simulink model "Ctrl_For_HRV_20260625"  (R2024b)
settings: Solver=ode4  StartTime=0.0  StopTime=22  FixedStep=0.02  RelTol=1e-3
InitFcn:
  | Parameter;
undefined symbols (not defined in the file or in its folder): CCI_DUI_AngleRate_Controller, CCI_DUI_FlowAngle_Controller, fhan, h_alpha, h_beta, h_miu, h_p, h_q, h_r, PNG_2026_6_23, r_alpha, r_beta, r_miu, r_p, r_q, r_r, xishu, xishu_D_0, xishu_L_0, xishu_l_0, xishu_m_0, xishu_n_0, xishu_Y_0
libraries: simulink x60
(part 2 of 8)

== system Ctrl_For_HRV_20260625/Vehicle_1/FlowAngle_Controller_v1 ==
  alpha_d : Inport
  beta_d : Inport  Port=2
  miu_d : Inport  Port=3
  Demux : Demux  Outputs=9
  From12 : From  Commented=on  GotoTag=dot_alpha_c  TagVisibility=global
  From13 : From  Commented=on  GotoTag=dot_beta_c  TagVisibility=global
  From14 : From  Commented=on  GotoTag=dot_miu_c  TagVisibility=global
  Goto6 : Goto  Commented=on  GotoTag=ddot_alpha_c  TagVisibility=global
  Goto7 : Goto  Commented=on  GotoTag=ddot_beta_c  TagVisibility=global
  Goto8 : Goto  Commented=on  GotoTag=ddot_miu_c  TagVisibility=global
  Interpreted MATLAB Function : MATLABFcn  MATLABFcn=CCI_DUI_FlowAngle_Controller(u(1),u(2),u(3),u(4),u(5),u(6),u(7),u(8),u(9),u(10),u(11),u(12),u(13),u(14),u(15),u(16),u(17),u(18))  OutputDimensions=9
  Mux : Mux  Inputs=18
  Mux1 : Mux  Inputs=3
  Mux2 : Mux  Inputs=3
  Scope_CCI_FlowAngle : Scope
  Scope_DUI_FlowAngle : Scope
  Scope_alpha_d : Scope
  Scope_beta_d : Scope
  Scope_miu_d : Scope
  TD_alpha : Subsystem
  TD_alpha2 : Subsystem
  TD_alpha3 : Subsystem  Commented=on
  TD_alpha4 : Subsystem  Commented=on
  TD_beta : Subsystem
  TD_beta1 : Subsystem
  TD_beta2 : Subsystem
  TD_dotalpha1 : Subsystem  Commented=on
  TD_miu : Subsystem
  p_d : Outport
  q_d : Outport  Port=2
  r_d : Outport  Port=3
  tag scope: alpha_c_v1=global, beta_c_v1=global, dot_alpha_c_v1=global, dot_beta_c_v1=global, dot_miu_c_v1=global, miu_c_v1=global
  wires:
  Demux/7 -> Mux2/1
  Demux/9 -> Mux2/3
  Demux/8 -> Mux2/2
  Mux2/1 -> Scope_DUI_FlowAngle/1
  Mux1/1 -> Scope_CCI_FlowAngle/1
  Demux/6 -> Mux1/3
  Demux/5 -> Mux1/2
  Demux/4 -> Mux1/1
  TD_alpha/1(alpha_c) -> Mux/13, [alpha_c_v1]
  TD_alpha4/1(ddot_miu_c) -> Goto8/1
  From14/1 -> TD_alpha4/1(dot_miu_c)
  TD_alpha3/1(ddot_beta_c) -> Goto7/1
  From13/1 -> TD_alpha3/1(dot_beta_c)
  TD_dotalpha1/1(ddot_alpha_c) -> Goto6/1
  From12/1 -> TD_dotalpha1/1(dot_alpha_c)
  [phi_miu_hat_v1] -> Mux/12
  [phi_beta_hat_v1] -> Mux/11
  [phi_alpha_hat_v1] -> Mux/10
  TD_miu/2(miu_c_dot) -> Mux/18, [dot_miu_c_v1]
  TD_miu/1(miu_c) -> Mux/17, [miu_c_v1]
  miu_d/1 -> TD_miu/1(miu_d), Scope_miu_d/1
  TD_beta/2(beta_c_dot) -> Mux/16, [dot_beta_c_v1]
  TD_beta/1(beta_c) -> Mux/15, [beta_c_v1]
  beta_d/1 -> TD_beta/1(beta_d), Scope_beta_d/1
  TD_alpha/2(alpha_c_dot) -> [dot_alpha_c_v1], Mux/14
  alpha_d/1 -> TD_alpha/1(alpha_d), Scope_alpha_d/1
  Demux/3 -> r_d/1
  Demux/2 -> q_d/1
  Demux/1 -> p_d/1
  Interpreted MATLAB Function/1 -> Demux/1
  Mux/1 -> Interpreted MATLAB Function/1
  [theta_v1] -> Mux/9
  [delta_a_v1] -> Mux/6
  [delta_e_v1] -> Mux/7
  [delta_r_v1] -> Mux/8
  [miu_noise_v1] -> Mux/5
  [beta_noise_v1] -> Mux/4
  [alpha_noise_v1] -> Mux/3
  [V_v1] -> Mux/2
  [H_v1] -> Mux/1

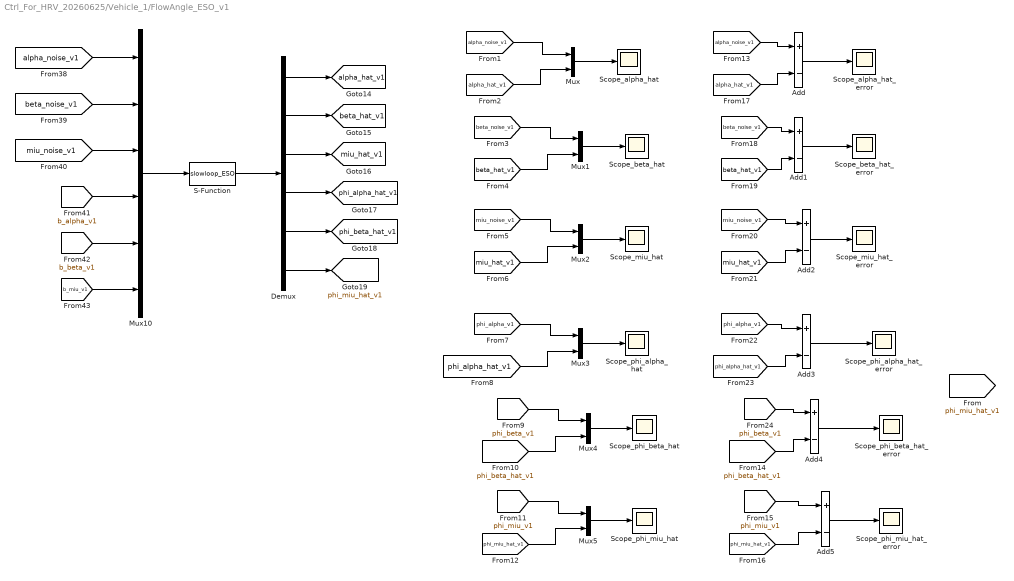
== system Ctrl_For_HRV_20260625/Vehicle_1/FlowAngle_ESO_v1 ==
  Add{,1..5} (6 alike) : Sum  Inputs=+-
  Demux : Demux  Outputs=6
  Mux{,1..5} (6 alike) : Mux  Inputs=2
  Mux10 : Mux  Inputs=6
  S-Function : S-Function  FunctionName=slowloop_ESO  SFunctionDeploymentMode=off  EnableBusSupport=off
  Scope_alpha_hat : Scope
  Scope_alpha_hat_error : Scope
  Scope_beta_hat : Scope
  Scope_beta_hat_error : Scope
  Scope_miu_hat : Scope
  Scope_miu_hat_error : Scope
  Scope_phi_alpha_hat : Scope
  Scope_phi_alpha_hat_error : Scope
  Scope_phi_beta_hat : Scope
  Scope_phi_beta_hat_error : Scope
  Scope_phi_miu_hat : Scope
  Scope_phi_miu_hat_error : Scope
  tag scope: alpha_hat_v1=global, beta_hat_v1=global, miu_hat_v1=global, phi_alpha_hat_v1=global, phi_beta_hat_v1=global, phi_miu_hat_v1=global
  wires:
  [phi_miu_hat_v1] -> Add5/2
  [phi_miu_v1] -> Add5/1
  Add5/1 -> Scope_phi_miu_hat_error/1
  Add4/1 -> Scope_phi_beta_hat_error/1
  [phi_beta_hat_v1] -> Add4/2
  [phi_beta_v1] -> Add4/1
  Add3/1 -> Scope_phi_alpha_hat_error/1
  [phi_alpha_hat_v1] -> Add3/2
  [phi_alpha_v1] -> Add3/1
  Add2/1 -> Scope_miu_hat_error/1
  [miu_hat_v1] -> Add2/2
  [miu_noise_v1] -> Add2/1
  Add1/1 -> Scope_beta_hat_error/1
  [beta_hat_v1] -> Add1/2
  [beta_noise_v1] -> Add1/1
  Add/1 -> Scope_alpha_hat_error/1
  [alpha_hat_v1] -> Add/2
  [alpha_noise_v1] -> Add/1
  Mux3/1 -> Scope_phi_alpha_hat/1
  [phi_alpha_v1] -> Mux3/1
  [phi_alpha_hat_v1] -> Mux3/2
  [phi_beta_v1] -> Mux4/1
  [phi_beta_hat_v1] -> Mux4/2
  Mux4/1 -> Scope_phi_beta_hat/1
  [phi_miu_v1] -> Mux5/1
  [phi_miu_hat_v1] -> Mux5/2
  Mux5/1 -> Scope_phi_miu_hat/1
  Mux2/1 -> Scope_miu_hat/1
  [miu_hat_v1] -> Mux2/2
  [miu_noise_v1] -> Mux2/1
  Mux1/1 -> Scope_beta_hat/1
  [beta_hat_v1] -> Mux1/2
  [beta_noise_v1] -> Mux1/1
  [alpha_hat_v1] -> Mux/2
  [alpha_noise_v1] -> Mux/1
  Mux/1 -> Scope_alpha_hat/1
  [b_miu_v1] -> Mux10/6
  [alpha_noise_v1] -> Mux10/1
  Demux/6 -> [phi_miu_hat_v1]
  Mux10/1 -> S-Function/1
  Demux/4 -> [phi_alpha_hat_v1]
  Demux/3 -> [miu_hat_v1]
  Demux/1 -> [alpha_hat_v1]
  Demux/5 -> [phi_beta_hat_v1]
  S-Function/1 -> Demux/1
  [b_alpha_v1] -> Mux10/4
  Demux/2 -> [beta_hat_v1]
  [beta_noise_v1] -> Mux10/2
  [miu_noise_v1] -> Mux10/3
  [b_beta_v1] -> Mux10/5

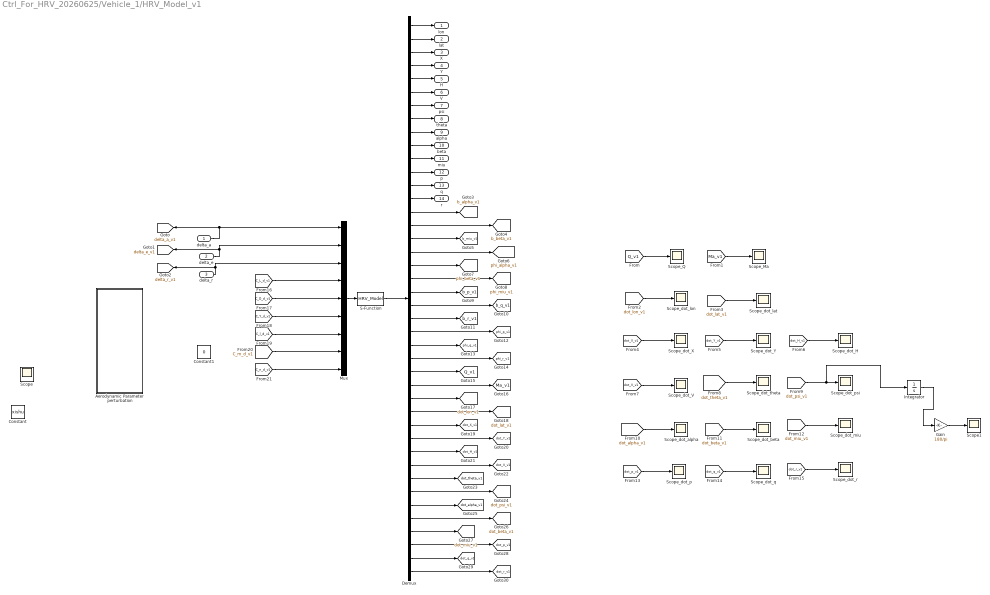
== system Ctrl_For_HRV_20260625/Vehicle_1/HRV_Model_v1 ==
  delta_a : Inport
  delta_e : Inport  Port=2
  delta_r : Inport  Port=3
  Aerodynamic Parameter perturbation : Subsystem
  Constant : Constant  Value=xishu  SampleTime=-1
  Constant1 : Constant  Value=0
  Demux : Demux  Outputs=14 + 12 + 2 + 14
  Gain : Gain  Gain=180/pi
  Integrator : Integrator  InitialCondition=[0 0 -900 -700 0 0 -0.0698131700797732 0 0 0 0 0 0 0 0 0 0 0 0 0 0 0 0 0 0 0 0 0 0 0 0 0 0 0 0 0 0 0 0 0 0 0]
  Mux : Mux  Inputs=9
  S-Function : S-Function  FunctionName=HRV_Model  SFunctionDeploymentMode=off  EnableBusSupport=off
  Scope : Scope
  Scope1 : Scope
  Scope_Ma : Scope
  Scope_Q : Scope
  Scope_dot_H : Scope
  Scope_dot_V : Scope
  Scope_dot_X : Scope
  Scope_dot_Y : Scope
  Scope_dot_alpha : Scope
  Scope_dot_beta : Scope
  Scope_dot_lat : Scope
  Scope_dot_lon : Scope
  Scope_dot_miu : Scope
  Scope_dot_p : Scope
  Scope_dot_psi : Scope
  Scope_dot_q : Scope
  Scope_dot_r : Scope
  Scope_dot_theta : Scope
  lon : Outport
  lat : Outport  Port=2
  X : Outport  Port=3
  Y : Outport  Port=4
  H : Outport  Port=5
  V : Outport  Port=6
  psi : Outport  Port=7
  theta : Outport  Port=8
  alpha : Outport  Port=9
  beta : Outport  Port=10
  miu : Outport  Port=11
  p : Outport  Port=12
  q : Outport  Port=13
  r : Outport  Port=14
  tag scope: Ma_v1=global, Q_v1=global, b_alpha_v1=global, b_beta_v1=global, b_miu_v1=global, b_p_v1=global, b_q_v1=global, b_r_v1=global, delta_a_v1=global, delta_e_v1=global, delta_r_v1=global, dot_H_v1=global, dot_V_v1=global, dot_X_v1=global, dot_Y_v1=global, dot_alpha_v1=global, dot_beta_v1=global, dot_lat_v1=global, dot_lon_v1=global, dot_miu_v1=global, dot_p_v1=global, dot_psi_v1=global, dot_q_v1=global, dot_r_v1=global, dot_theta_v1=global, phi_alpha_v1=global, phi_beta_v1=global, phi_miu_v1=global, phi_p_v1=global, phi_q_v1=global, phi_r_v1=global
  wires:
  Gain/1 -> Scope1/1
  Integrator/1 -> Gain/1
  [C_n_d_v1] -> Mux/9
  [C_m_d_v1] -> Mux/8
  [C_l_d_v1] -> Mux/7
  [C_Y_d_v1] -> Mux/6
  [C_D_d_v1] -> Mux/5
  [C_L_d_v1] -> Mux/4
  [dot_p_v1] -> Scope_dot_p/1
  [dot_q_v1] -> Scope_dot_q/1
  [dot_r_v1] -> Scope_dot_r/1
  [dot_miu_v1] -> Scope_dot_miu/1
  [dot_beta_v1] -> Scope_dot_beta/1
  [dot_alpha_v1] -> Scope_dot_alpha/1
  [dot_psi_v1] -> Scope_dot_psi/1, Integrator/1
  [dot_theta_v1] -> Scope_dot_theta/1
  [dot_V_v1] -> Scope_dot_V/1
  [dot_H_v1] -> Scope_dot_H/1
  [dot_Y_v1] -> Scope_dot_Y/1
  [dot_X_v1] -> Scope_dot_X/1
  [dot_lat_v1] -> Scope_dot_lat/1
  [dot_lon_v1] -> Scope_dot_lon/1
  [Ma_v1] -> Scope_Ma/1
  [Q_v1] -> Scope_Q/1
  Demux/42 -> [dot_r_v1]
  Demux/41 -> [dot_q_v1]
  Demux/40 -> [dot_p_v1]
  Demux/38 -> [dot_beta_v1]
  Demux/39 -> [dot_miu_v1]
  Demux/33 -> [dot_H_v1]
  Demux/35 -> [dot_theta_v1]
  Demux/34 -> [dot_V_v1]
  Demux/36 -> [dot_psi_v1]
  Demux/37 -> [dot_alpha_v1]
  Demux/32 -> [dot_Y_v1]
  Demux/31 -> [dot_X_v1]
  Demux/29 -> [dot_lon_v1]
  Demux/30 -> [dot_lat_v1]
  Demux/28 -> [Ma_v1]
  Demux/27 -> [Q_v1]
  Demux/26 -> [phi_r_v1]
  Demux/25 -> [phi_q_v1]
  Demux/24 -> [phi_p_v1]
  Demux/23 -> [b_r_v1]
  Demux/19 -> [phi_beta_v1]
  Demux/20 -> [phi_miu_v1]
  Demux/22 -> [b_q_v1]
  Demux/21 -> [b_p_v1]
  Demux/17 -> [b_miu_v1]
  Demux/18 -> [phi_alpha_v1]
  Demux/16 -> [b_beta_v1]
  Demux/15 -> [b_alpha_v1]
  Demux/4 -> Y/1
  delta_a/1 -> Mux/1, [delta_a_v1]
  Demux/13 -> q/1
  delta_r/1 -> Mux/3, [delta_r_v1]
  Demux/14 -> r/1
  Demux/6 -> V/1
  delta_e/1 -> Mux/2, [delta_e_v1]
  Demux/5 -> H/1
  Demux/12 -> p/1
  Demux/9 -> alpha/1
  Demux/10 -> beta/1
  Demux/11 -> miu/1
  Demux/7 -> psi/1
  Demux/3 -> X/1
  Demux/2 -> lat/1
  Demux/1 -> lon/1
  S-Function/1 -> Demux/1
  Mux/1 -> S-Function/1
  Demux/8 -> theta/1

== system Ctrl_For_HRV_20260625/Vehicle_1/PNG ==
  Delay : Delay  DelayLength=1
  Demux : Demux  Outputs=3
  MATLAB Function : MATLAB Function  TreatAsAtomicUnit=on
  MATLAB Function1 : MATLAB Function  TreatAsAtomicUnit=on  SystemSampleTime=0.02
  MATLAB Function2 : MATLAB Function  TreatAsAtomicUnit=on
  Mux : Mux  Inputs=7+2
  PNG : MATLABFcn  MATLABFcn=PNG_2026_6_23(u)  OutputDimensions=3
  Scope{,1..4} (5 alike) : Scope
  Scope5 : Scope  NumInputPorts=2
  tag scope: alpha_cmd=global, f_psi=global, miu_cmd=global
  wires:
  Delay/1 -> MATLAB Function1/6(miu_last)
  [theta] -> Mux/9
  [f_psi] -> Mux/8
  MATLAB Function2/1(f_psi) -> [f_psi]
  [H] -> MATLAB Function2/5(H)
  [lat] -> MATLAB Function2/4(lat)
  [psi] -> MATLAB Function2/3(psi)
  [theta] -> MATLAB Function2/2(theta)
  [V] -> MATLAB Function2/1(V)
  Demux/3 -> Scope5/1
  [Q] -> Mux/7
  MATLAB Function1/2(miu_cmd) -> [miu_cmd], Scope3/1, Delay/1
  MATLAB Function1/1(alpha_cmd) -> [alpha_cmd], Scope2/1
  [Ma] -> MATLAB Function1/5(Ma)
  [H] -> MATLAB Function1/4(H)
  [Q] -> MATLAB Function1/3(Q)
  [nz_cmd] -> MATLAB Function1/2(nz_cmd)
  [ny_cmd] -> MATLAB Function1/1(ny_cmd)
  [nz_cmd] -> Scope1/1
  [ny_cmd] -> Scope/1
  Demux/2 -> [nz_cmd], Scope5/2
  Demux/1 -> [ny_cmd]
  PNG/1 -> Demux/1
  [V_target] -> Mux/6
  [Position_target] -> Mux/5
  MATLAB Function/1(v) -> Mux/4, Scope4/1
  [psi] -> MATLAB Function/3(psi)
  [theta] -> MATLAB Function/2(theta)
  [V] -> MATLAB Function/1(V)
  [H] -> Mux/3
  [Y] -> Mux/2
  [X] -> Mux/1
  Mux/1 -> PNG/1

== system Ctrl_For_HRV_20260625/Vehicle_1/actuator1_v1 ==
  delta_e_d : Inport
  Gain : Gain  Gain=50
  Integrator : Integrator
  Saturation : Saturate  UpperLimit=90  LowerLimit=-90
  Saturation1 : Saturate  UpperLimit=30  LowerLimit=-30
  Sum : Sum  Inputs=|+-
  delta_e : Outport
  wires:
  Saturation/1 -> Integrator/1
  Sum/1 -> Gain/1
  Integrator/1 -> Saturation1/1, Sum/2
  delta_e_d/1 -> Sum/1
  Gain/1 -> Saturation/1
  Saturation1/1 -> delta_e/1

== system Ctrl_For_HRV_20260625/Vehicle_1/actuator2_v1 ==
  delta_r_d : Inport
  Gain : Gain  Gain=50
  Integrator : Integrator
  Saturation : Saturate  UpperLimit=90  LowerLimit=-90
  Saturation1 : Saturate  UpperLimit=30  LowerLimit=-30
  Sum : Sum  Inputs=|+-
  delta_r : Outport
  wires:
  Saturation1/1 -> delta_r/1
  Gain/1 -> Saturation/1
  delta_r_d/1 -> Sum/1
  Integrator/1 -> Sum/2, Saturation1/1
  Sum/1 -> Gain/1
  Saturation/1 -> Integrator/1

== system Ctrl_For_HRV_20260625/Vehicle_1/actuator_v1 ==
  delta_a_d : Inport
  Gain : Gain  Gain=50
  Integrator : Integrator
  Saturation : Saturate  UpperLimit=90  LowerLimit=-90
  Saturation1 : Saturate  UpperLimit=30  LowerLimit=-30
  Sum : Sum  Inputs=|+-
  delta_a : Outport
  wires:
  Saturation1/1 -> delta_a/1
  Gain/1 -> Saturation/1
  delta_a_d/1 -> Sum/1
  Integrator/1 -> Sum/2, Saturation1/1
  Sum/1 -> Gain/1
  Saturation/1 -> Integrator/1

== system Ctrl_For_HRV_20260625/Vehicle_2/AngleRate_Controller_v2 ==
  p_d : Inport
  q_d : Inport  Port=2
  r_d : Inport  Port=3
  Demux : Demux  Outputs=9
  Interpreted MATLAB Function : MATLABFcn  MATLABFcn=CCI_DUI_AngleRate_Controller(u(1),u(2),u(3),u(4),u(5),u(6),u(7),u(8),u(9),u(10),u(11),u(12),u(13),u(14),u(15),u(16),u(17),u(18),u(19),u(20),u(21),u(22),u(23))  OutputDimensions=9
  Mux : Mux  Inputs=23
  Mux1 : Mux  Inputs=3
  Mux2 : Mux  Inputs=3
  Scope2 : Scope
  Scope_CCI_AngleRate : Scope
  Scope_DUI_AngleRate : Scope
  Scope_p_d : Scope
  Scope_q_d : Scope
  Scope_r_d : Scope
  TD_p : Subsystem
  TD_q : Subsystem
  TD_r : Subsystem
  delta_a_d : Outport
  delta_e_d : Outport  Port=2
  delta_r_d : Outport  Port=3
  tag scope: delta_a_d_v2=global, delta_e_d_v2=global, delta_r_d_v2=global, p_c_v2=global, q_c_v2=global, r_c_v2=global
  wires:
  Mux2/1 -> Scope_DUI_AngleRate/1
  Demux/9 -> Mux2/3
  Demux/8 -> Mux2/2
  Demux/7 -> Mux2/1
  Mux1/1 -> Scope_CCI_AngleRate/1
  Demux/6 -> Mux1/3
  Demux/5 -> Mux1/2
  Demux/4 -> Mux1/1
  [miu_c_v2] -> Mux/23
  [beta_c_v2] -> Mux/22
  [alpha_c_v2] -> Mux/21
  [phi_r_hat_v2] -> Mux/14
  [phi_q_hat_v2] -> Mux/13
  [phi_p_hat_v2] -> Mux/12
  p_d/1 -> TD_p/1(p_d), Scope_p_d/1
  q_d/1 -> TD_q/1(q_d), Scope_q_d/1
  Demux/1 -> delta_a_d/1, [delta_a_d_v2]
  Demux/2 -> delta_e_d/1, [delta_e_d_v2]
  r_d/1 -> TD_r/1(r_d), Scope_r_d/1
  Demux/3 -> [delta_r_d_v2], delta_r_d/1
  TD_p/1(p_c) -> Mux/15, [p_c_v2]
  [delta_e_v2] -> Mux/7
  [delta_r_v2] -> Mux/8
  [delta_a_v2] -> Mux/6
  Interpreted MATLAB Function/1 -> Demux/1
  Mux/1 -> Interpreted MATLAB Function/1
  [alpha_noise_v2] -> Mux/3
  [V_v2] -> Mux/2
  [p_noise_v2] -> Mux/9
  [H_v2] -> Mux/1
  [r_noise_v2] -> Mux/11
  TD_r/2(r_c_dot) -> Mux/20
  TD_q/1(q_c) -> Mux/17, [q_c_v2]
  [q_noise_v2] -> Mux/10
  TD_q/2(q_c_dot) -> Mux/18
  TD_p/2(p_c_dot) -> Mux/16
  TD_r/1(r_c) -> Mux/19, [r_c_v2]
  [beta_noise_v2] -> Mux/4
  [miu_noise_v2] -> Mux/5

== system Ctrl_For_HRV_20260625/Vehicle_2/AngleRate_ESO_v2 ==
  Add{,1..5} (6 alike) : Sum  Inputs=+-
  Demux : Demux  Outputs=6
  Mux{,1..5} (6 alike) : Mux  Inputs=2
  Mux10 : Mux  Inputs=6
  S-Function : S-Function  FunctionName=fastloop_ESO  SFunctionDeploymentMode=off  EnableBusSupport=off
  Scope_p_hat : Scope
  Scope_p_hat_error : Scope
  Scope_phi_p_hat : Scope
  Scope_phi_p_hat_error : Scope
  Scope_phi_q_hat : Scope
  Scope_phi_q_hat_error : Scope
  Scope_phi_r_hat : Scope
  Scope_phi_r_hat_error : Scope
  Scope_q_hat : Scope
  Scope_q_hat_error : Scope
  Scope_r_hat : Scope
  Scope_r_hat_error : Scope
  tag scope: p_hat_v2=global, phi_p_hat_v2=global, phi_q_hat_v2=global, phi_r_hat_v2=global, q_hat_v2=global, r_hat_v2=global
  wires:
  Add5/1 -> Scope_phi_r_hat_error/1
  [phi_r_hat_v2] -> Add5/2
  [phi_r_v2] -> Add5/1
  Add4/1 -> Scope_phi_q_hat_error/1
  [phi_q_hat_v2] -> Add4/2
  [phi_q_v2] -> Add4/1
  Add3/1 -> Scope_phi_p_hat_error/1
  [phi_p_hat_v2] -> Add3/2
  [phi_p_v2] -> Add3/1
  Add2/1 -> Scope_r_hat_error/1
  [r_hat_v2] -> Add2/2
  [r_noise_v2] -> Add2/1
  Add1/1 -> Scope_q_hat_error/1
  [q_hat_v2] -> Add1/2
  [q_noise_v2] -> Add1/1
  Add/1 -> Scope_p_hat_error/1
  [p_hat_v2] -> Add/2
  [p_noise_v2] -> Add/1
  Mux3/1 -> Scope_phi_p_hat/1
  [phi_p_v2] -> Mux3/1
  [phi_p_hat_v2] -> Mux3/2
  [phi_q_v2] -> Mux4/1
  [phi_q_hat_v2] -> Mux4/2
  Mux4/1 -> Scope_phi_q_hat/1
  [phi_r_v2] -> Mux5/1
  [phi_r_hat_v2] -> Mux5/2
  Mux5/1 -> Scope_phi_r_hat/1
  Mux2/1 -> Scope_r_hat/1
  [r_hat_v2] -> Mux2/2
  [r_noise_v2] -> Mux2/1
  Mux1/1 -> Scope_q_hat/1
  [q_hat_v2] -> Mux1/2
  [q_noise_v2] -> Mux1/1
  [p_hat_v2] -> Mux/2
  [p_noise_v2] -> Mux/1
  Mux/1 -> Scope_p_hat/1
  [b_r_v2] -> Mux10/6
  [p_noise_v2] -> Mux10/1
  Demux/6 -> [phi_r_hat_v2]
  Mux10/1 -> S-Function/1
  Demux/4 -> [phi_p_hat_v2]
  Demux/3 -> [r_hat_v2]
  Demux/1 -> [p_hat_v2]
  Demux/5 -> [phi_q_hat_v2]
  S-Function/1 -> Demux/1
  [b_p_v2] -> Mux10/4
  Demux/2 -> [q_hat_v2]
  [q_noise_v2] -> Mux10/2
  [r_noise_v2] -> Mux10/3
  [b_q_v2] -> Mux10/5

== system Ctrl_For_HRV_20260625/Vehicle_2/Error_Model ==
  Delay : Delay  DelayLength=1
  Delay1 : Delay  DelayLength=1
  Delay2 : Delay  DelayLength=1
  Demux : Demux  Outputs=9
  Mux : Mux  Inputs=33
  S-Function : S-Function  FunctionName=Error_Model  SFunctionDeploymentMode=off  EnableBusSupport=off
  TD_alpha1 : Subsystem
  TD_alpha2 : Subsystem
  TD_alpha3 : Subsystem
  tag scope: dot_e_wd_1=global, dot_e_wd_2=global, dot_e_wd_3=global, e_alpha=global, e_beta=global, e_miu=global, e_w_1=global, e_w_2=global, e_w_3=global, e_wd_1=global, e_wd_2=global, e_wd_3=global
  wires:
  [theta] -> Mux/33
  [r] -> Mux/32
  [q] -> Mux/31
  [p] -> Mux/30
  [miu] -> Mux/29
  [beta] -> Mux/28
  [alpha] -> Mux/27
  [delta_r] -> Mux/3
  [delta_e] -> Mux/2
  [delta_a] -> Mux/1
  [dot_e_wd_3] -> Mux/26
  [dot_e_wd_2] -> Mux/25
  [dot_e_wd_1] -> Mux/24
  TD_alpha3/1(dot_e_wd_3) -> [dot_e_wd_3]
  [e_wd_3] -> TD_alpha3/1(e_wd_3)
  [e_wd_2] -> TD_alpha2/1(e_wd_2)
  TD_alpha2/1(dot_e_wd_2) -> [dot_e_wd_2]
  TD_alpha1/1(dot_e_wd_1) -> [dot_e_wd_1]
  [e_wd_1] -> TD_alpha1/1(e_wd_1)
  Delay2/1 -> Mux/23
  [e_wd_3] -> Delay2/1
  [e_wd_2] -> Delay1/1
  Delay1/1 -> Mux/22
  Delay/1 -> Mux/21
  [e_wd_1] -> Delay/1
  Demux/7 -> [e_wd_1]
  Demux/8 -> [e_wd_2]
  Demux/9 -> [e_wd_3]
  Demux/6 -> [e_w_3]
  Demux/5 -> [e_w_2]
  Demux/4 -> [e_w_1]
  Demux/3 -> [e_miu]
  Demux/2 -> [e_beta]
  Demux/1 -> [e_alpha]
  S-Function/1 -> Demux/1
  [ddot_miu_c] -> Mux/20
  [ddot_beta_c] -> Mux/19
  [ddot_alpha_c] -> Mux/18
  [dot_alpha_c] -> Mux/15
  [dot_beta_c] -> Mux/16
  [dot_miu_c] -> Mux/17
  [miu_c] -> Mux/14
  [beta_c] -> Mux/13
  [alpha_c] -> Mux/12
  [V] -> Mux/11
  [H] -> Mux/10
  [C_m_d] -> Mux/8
  [C_n_d] -> Mux/9
  [C_Y_d] -> Mux/6
  [C_L_d] -> Mux/4
  [C_D_d] -> Mux/5
  [C_l_d] -> Mux/7
  Mux/1 -> S-Function/1

== system Ctrl_For_HRV_20260625/Vehicle_2/FlowAngle_Controller_v2 ==
  alpha_d : Inport
  beta_d : Inport  Port=2
  miu_d : Inport  Port=3
  Demux : Demux  Outputs=9
  From12 : From  Commented=on  GotoTag=dot_alpha_c  TagVisibility=global
  From13 : From  Commented=on  GotoTag=dot_beta_c  TagVisibility=global
  From14 : From  Commented=on  GotoTag=dot_miu_c  TagVisibility=global
  Goto6 : Goto  Commented=on  GotoTag=ddot_alpha_c  TagVisibility=global
  Goto7 : Goto  Commented=on  GotoTag=ddot_beta_c  TagVisibility=global
  Goto8 : Goto  Commented=on  GotoTag=ddot_miu_c  TagVisibility=global
  Interpreted MATLAB Function : MATLABFcn  MATLABFcn=CCI_DUI_FlowAngle_Controller(u(1),u(2),u(3),u(4),u(5),u(6),u(7),u(8),u(9),u(10),u(11),u(12),u(13),u(14),u(15),u(16),u(17),u(18))  OutputDimensions=9
  Mux : Mux  Inputs=18
  Mux1 : Mux  Inputs=3
  Mux2 : Mux  Inputs=3
  Scope_CCI_FlowAngle : Scope
  Scope_DUI_FlowAngle : Scope
  Scope_alpha_d : Scope
  Scope_beta_d : Scope
  Scope_miu_d : Scope
  TD_alpha : Subsystem
  TD_alpha2 : Subsystem
  TD_alpha3 : Subsystem  Commented=on
  TD_alpha4 : Subsystem  Commented=on
  TD_beta : Subsystem
  TD_beta1 : Subsystem
  TD_beta2 : Subsystem
  TD_dotalpha1 : Subsystem  Commented=on
  TD_miu : Subsystem
  p_d : Outport
  q_d : Outport  Port=2
  r_d : Outport  Port=3
  tag scope: alpha_c_v2=global, beta_c_v2=global, dot_alpha_c_v2=global, dot_beta_c_v2=global, dot_miu_c_v2=global, miu_c_v2=global
  wires:
  Demux/7 -> Mux2/1
  Demux/9 -> Mux2/3
  Demux/8 -> Mux2/2
  Mux2/1 -> Scope_DUI_FlowAngle/1
  Mux1/1 -> Scope_CCI_FlowAngle/1
  Demux/6 -> Mux1/3
  Demux/5 -> Mux1/2
  Demux/4 -> Mux1/1
  TD_alpha/1(alpha_c) -> Mux/13, [alpha_c_v2]
  TD_alpha4/1(ddot_miu_c) -> Goto8/1
  From14/1 -> TD_alpha4/1(dot_miu_c)
  TD_alpha3/1(ddot_beta_c) -> Goto7/1
  From13/1 -> TD_alpha3/1(dot_beta_c)
  TD_dotalpha1/1(ddot_alpha_c) -> Goto6/1
  From12/1 -> TD_dotalpha1/1(dot_alpha_c)
  [phi_miu_hat_v2] -> Mux/12
  [phi_beta_hat_v2] -> Mux/11
  [phi_alpha_hat_v2] -> Mux/10
  TD_miu/2(miu_c_dot) -> Mux/18, [dot_miu_c_v2]
  TD_miu/1(miu_c) -> Mux/17, [miu_c_v2]
  miu_d/1 -> TD_miu/1(miu_d), Scope_miu_d/1
  TD_beta/2(beta_c_dot) -> Mux/16, [dot_beta_c_v2]
  TD_beta/1(beta_c) -> Mux/15, [beta_c_v2]
  beta_d/1 -> TD_beta/1(beta_d), Scope_beta_d/1
  TD_alpha/2(alpha_c_dot) -> [dot_alpha_c_v2], Mux/14
  alpha_d/1 -> TD_alpha/1(alpha_d), Scope_alpha_d/1
  Demux/3 -> r_d/1
  Demux/2 -> q_d/1
  Demux/1 -> p_d/1
  Interpreted MATLAB Function/1 -> Demux/1
  Mux/1 -> Interpreted MATLAB Function/1
  [theta_v2] -> Mux/9
  [delta_a_v2] -> Mux/6
  [delta_e_v2] -> Mux/7
  [delta_r_v2] -> Mux/8
  [miu_noise_v2] -> Mux/5
  [beta_noise_v2] -> Mux/4
  [alpha_noise_v2] -> Mux/3
  [V_v2] -> Mux/2
  [H_v2] -> Mux/1

== system Ctrl_For_HRV_20260625/Vehicle_2/FlowAngle_ESO_v2 ==
  Add{,1..5} (6 alike) : Sum  Inputs=+-
  Demux : Demux  Outputs=6
  Mux{,1..5} (6 alike) : Mux  Inputs=2
  Mux10 : Mux  Inputs=6
  S-Function : S-Function  FunctionName=slowloop_ESO  SFunctionDeploymentMode=off  EnableBusSupport=off
  Scope_alpha_hat : Scope
  Scope_alpha_hat_error : Scope
  Scope_beta_hat : Scope
  Scope_beta_hat_error : Scope
  Scope_miu_hat : Scope
  Scope_miu_hat_error : Scope
  Scope_phi_alpha_hat : Scope
  Scope_phi_alpha_hat_error : Scope
  Scope_phi_beta_hat : Scope
  Scope_phi_beta_hat_error : Scope
  Scope_phi_miu_hat : Scope
  Scope_phi_miu_hat_error : Scope
  tag scope: alpha_hat_v2=global, beta_hat_v2=global, miu_hat_v2=global, phi_alpha_hat_v2=global, phi_beta_hat_v2=global, phi_miu_hat_v2=global
  wires:
  [phi_miu_hat_v2] -> Add5/2
  [phi_miu_v2] -> Add5/1
  Add5/1 -> Scope_phi_miu_hat_error/1
  Add4/1 -> Scope_phi_beta_hat_error/1
  [phi_beta_hat_v2] -> Add4/2
  [phi_beta_v2] -> Add4/1
  Add3/1 -> Scope_phi_alpha_hat_error/1
  [phi_alpha_hat_v2] -> Add3/2
  [phi_alpha_v2] -> Add3/1
  Add2/1 -> Scope_miu_hat_error/1
  [miu_hat_v2] -> Add2/2
  [miu_noise_v2] -> Add2/1
  Add1/1 -> Scope_beta_hat_error/1
  [beta_hat_v2] -> Add1/2
  [beta_noise_v2] -> Add1/1
  Add/1 -> Scope_alpha_hat_error/1
  [alpha_hat_v2] -> Add/2
  [alpha_noise_v2] -> Add/1
  Mux3/1 -> Scope_phi_alpha_hat/1
  [phi_alpha_v2] -> Mux3/1
  [phi_alpha_hat_v2] -> Mux3/2
  [phi_beta_v2] -> Mux4/1
  [phi_beta_hat_v2] -> Mux4/2
  Mux4/1 -> Scope_phi_beta_hat/1
  [phi_miu_v2] -> Mux5/1
  [phi_miu_hat_v2] -> Mux5/2
  Mux5/1 -> Scope_phi_miu_hat/1
  Mux2/1 -> Scope_miu_hat/1
  [miu_hat_v2] -> Mux2/2
  [miu_noise_v2] -> Mux2/1
  Mux1/1 -> Scope_beta_hat/1
  [beta_hat_v2] -> Mux1/2
  [beta_noise_v2] -> Mux1/1
  [alpha_hat_v2] -> Mux/2
  [alpha_noise_v2] -> Mux/1
  Mux/1 -> Scope_alpha_hat/1
  [b_miu_v2] -> Mux10/6
  [alpha_noise_v2] -> Mux10/1
  Demux/6 -> [phi_miu_hat_v2]
  Mux10/1 -> S-Function/1
  Demux/4 -> [phi_alpha_hat_v2]
  Demux/3 -> [miu_hat_v2]
  Demux/1 -> [alpha_hat_v2]
  Demux/5 -> [phi_beta_hat_v2]
  S-Function/1 -> Demux/1
  [b_alpha_v2] -> Mux10/4
  Demux/2 -> [beta_hat_v2]
  [beta_noise_v2] -> Mux10/2
  [miu_noise_v2] -> Mux10/3
  [b_beta_v2] -> Mux10/5

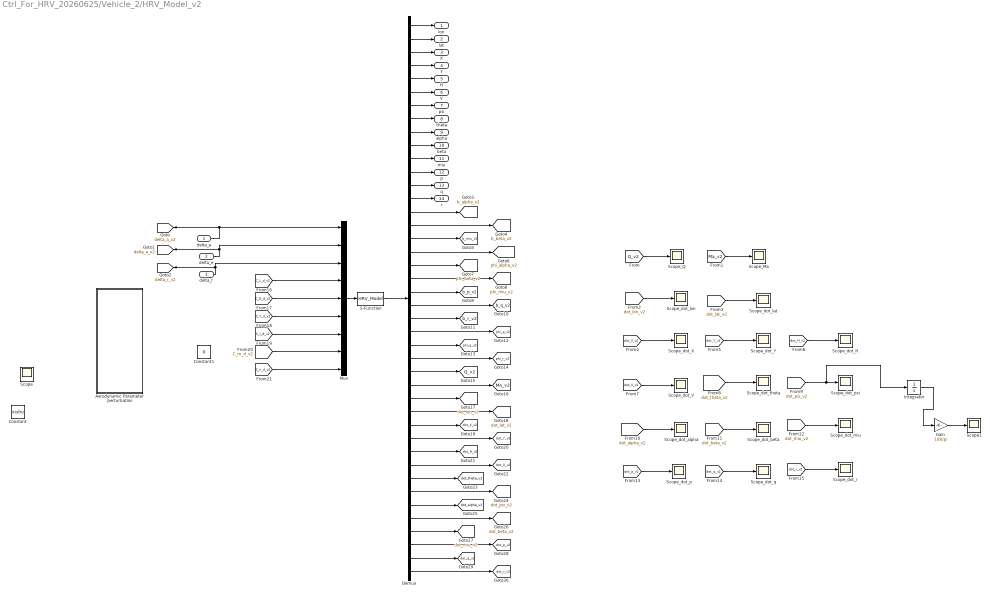
== system Ctrl_For_HRV_20260625/Vehicle_2/HRV_Model_v2 ==
  delta_a : Inport
  delta_e : Inport  Port=2
  delta_r : Inport  Port=3
  Aerodynamic Parameter perturbation : Subsystem
  Constant : Constant  Value=xishu  SampleTime=-1
  Constant1 : Constant  Value=0
  Demux : Demux  Outputs=14 + 12 + 2 + 14
  Gain : Gain  Gain=180/pi
  Integrator : Integrator  InitialCondition=[0 0 -450 -350 0 0 -0.0349065850398866 0 0 0 0 0 0 0 0 0 0 0 0 0 0 0 0 0 0 0 0 0 0 0 0 0 0 0 0 0 0 0 0 0 0 0]
  Mux : Mux  Inputs=9
  S-Function : S-Function  FunctionName=HRV_Model  SFunctionDeploymentMode=off  EnableBusSupport=off
  Scope : Scope
  Scope1 : Scope
  Scope_Ma : Scope
  Scope_Q : Scope
  Scope_dot_H : Scope
  Scope_dot_V : Scope
  Scope_dot_X : Scope
  Scope_dot_Y : Scope
  Scope_dot_alpha : Scope
  Scope_dot_beta : Scope
  Scope_dot_lat : Scope
  Scope_dot_lon : Scope
  Scope_dot_miu : Scope
  Scope_dot_p : Scope
  Scope_dot_psi : Scope
  Scope_dot_q : Scope
  Scope_dot_r : Scope
  Scope_dot_theta : Scope
  lon : Outport
  lat : Outport  Port=2
  X : Outport  Port=3
  Y : Outport  Port=4
  H : Outport  Port=5
  V : Outport  Port=6
  psi : Outport  Port=7
  theta : Outport  Port=8
  alpha : Outport  Port=9
  beta : Outport  Port=10
  miu : Outport  Port=11
  p : Outport  Port=12
  q : Outport  Port=13
  r : Outport  Port=14
  tag scope: Ma_v2=global, Q_v2=global, b_alpha_v2=global, b_beta_v2=global, b_miu_v2=global, b_p_v2=global, b_q_v2=global, b_r_v2=global, delta_a_v2=global, delta_e_v2=global, delta_r_v2=global, dot_H_v2=global, dot_V_v2=global, dot_X_v2=global, dot_Y_v2=global, dot_alpha_v2=global, dot_beta_v2=global, dot_lat_v2=global, dot_lon_v2=global, dot_miu_v2=global, dot_p_v2=global, dot_psi_v2=global, dot_q_v2=global, dot_r_v2=global, dot_theta_v2=global, phi_alpha_v2=global, phi_beta_v2=global, phi_miu_v2=global, phi_p_v2=global, phi_q_v2=global, phi_r_v2=global
  wires:
  Gain/1 -> Scope1/1
  Integrator/1 -> Gain/1
  [C_n_d_v2] -> Mux/9
  [C_m_d_v2] -> Mux/8
  [C_l_d_v2] -> Mux/7
  [C_Y_d_v2] -> Mux/6
  [C_D_d_v2] -> Mux/5
  [C_L_d_v2] -> Mux/4
  [dot_p_v2] -> Scope_dot_p/1
  [dot_q_v2] -> Scope_dot_q/1
  [dot_r_v2] -> Scope_dot_r/1
  [dot_miu_v2] -> Scope_dot_miu/1
  [dot_beta_v2] -> Scope_dot_beta/1
  [dot_alpha_v2] -> Scope_dot_alpha/1
  [dot_psi_v2] -> Scope_dot_psi/1, Integrator/1
  [dot_theta_v2] -> Scope_dot_theta/1
  [dot_V_v2] -> Scope_dot_V/1
  [dot_H_v2] -> Scope_dot_H/1
  [dot_Y_v2] -> Scope_dot_Y/1
  [dot_X_v2] -> Scope_dot_X/1
  [dot_lat_v2] -> Scope_dot_lat/1
  [dot_lon_v2] -> Scope_dot_lon/1
  [Ma_v2] -> Scope_Ma/1
  [Q_v2] -> Scope_Q/1
  Demux/42 -> [dot_r_v2]
  Demux/41 -> [dot_q_v2]
  Demux/40 -> [dot_p_v2]
  Demux/38 -> [dot_beta_v2]
  Demux/39 -> [dot_miu_v2]
  Demux/33 -> [dot_H_v2]
  Demux/35 -> [dot_theta_v2]
  Demux/34 -> [dot_V_v2]
  Demux/36 -> [dot_psi_v2]
  Demux/37 -> [dot_alpha_v2]
  Demux/32 -> [dot_Y_v2]
  Demux/31 -> [dot_X_v2]
  Demux/29 -> [dot_lon_v2]
  Demux/30 -> [dot_lat_v2]
  Demux/28 -> [Ma_v2]
  Demux/27 -> [Q_v2]
  Demux/26 -> [phi_r_v2]
  Demux/25 -> [phi_q_v2]
  Demux/24 -> [phi_p_v2]
  Demux/23 -> [b_r_v2]
  Demux/19 -> [phi_beta_v2]
  Demux/20 -> [phi_miu_v2]
  Demux/22 -> [b_q_v2]
  Demux/21 -> [b_p_v2]
  Demux/17 -> [b_miu_v2]
  Demux/18 -> [phi_alpha_v2]
  Demux/16 -> [b_beta_v2]
  Demux/15 -> [b_alpha_v2]
  Demux/4 -> Y/1
  delta_a/1 -> Mux/1, [delta_a_v2]
  Demux/13 -> q/1
  delta_r/1 -> Mux/3, [delta_r_v2]
  Demux/14 -> r/1
  Demux/6 -> V/1
  delta_e/1 -> Mux/2, [delta_e_v2]
  Demux/5 -> H/1
  Demux/12 -> p/1
  Demux/9 -> alpha/1
  Demux/10 -> beta/1
  Demux/11 -> miu/1
  Demux/7 -> psi/1
  Demux/3 -> X/1
  Demux/2 -> lat/1
  Demux/1 -> lon/1
  S-Function/1 -> Demux/1
  Mux/1 -> S-Function/1
  Demux/8 -> theta/1

== system Ctrl_For_HRV_20260625/Vehicle_2/PNG ==
  Delay : Delay  DelayLength=1
  Demux : Demux  Outputs=3
  MATLAB Function : MATLAB Function  TreatAsAtomicUnit=on
  MATLAB Function1 : MATLAB Function  TreatAsAtomicUnit=on  SystemSampleTime=0.02
  MATLAB Function2 : MATLAB Function  TreatAsAtomicUnit=on
  Mux : Mux  Inputs=7+2
  PNG : MATLABFcn  MATLABFcn=PNG_2026_6_23(u)  OutputDimensions=3
  Scope{,1..4} (5 alike) : Scope
  Scope5 : Scope  NumInputPorts=2
  tag scope: alpha_cmd=global, f_psi=global, miu_cmd=global
  wires:
  Delay/1 -> MATLAB Function1/6(miu_last)
  [theta] -> Mux/9
  [f_psi] -> Mux/8
  MATLAB Function2/1(f_psi) -> [f_psi]
  [H] -> MATLAB Function2/5(H)
  [lat] -> MATLAB Function2/4(lat)
  [psi] -> MATLAB Function2/3(psi)
  [theta] -> MATLAB Function2/2(theta)
  [V] -> MATLAB Function2/1(V)
  Demux/3 -> Scope5/1
  [Q] -> Mux/7
  MATLAB Function1/2(miu_cmd) -> [miu_cmd], Scope3/1, Delay/1
  MATLAB Function1/1(alpha_cmd) -> [alpha_cmd], Scope2/1
  [Ma] -> MATLAB Function1/5(Ma)
  [H] -> MATLAB Function1/4(H)
  [Q] -> MATLAB Function1/3(Q)
  [nz_cmd] -> MATLAB Function1/2(nz_cmd)
  [ny_cmd] -> MATLAB Function1/1(ny_cmd)
  [nz_cmd] -> Scope1/1
  [ny_cmd] -> Scope/1
  Demux/2 -> [nz_cmd], Scope5/2
  Demux/1 -> [ny_cmd]
  PNG/1 -> Demux/1
  [V_target] -> Mux/6
  [Position_target] -> Mux/5
  MATLAB Function/1(v) -> Mux/4, Scope4/1
  [psi] -> MATLAB Function/3(psi)
  [theta] -> MATLAB Function/2(theta)
  [V] -> MATLAB Function/1(V)
  [H] -> Mux/3
  [Y] -> Mux/2
  [X] -> Mux/1
  Mux/1 -> PNG/1

== system Ctrl_For_HRV_20260625/Vehicle_2/actuator1_v2 ==
  delta_e_d : Inport
  Gain : Gain  Gain=50
  Integrator : Integrator
  Saturation : Saturate  UpperLimit=90  LowerLimit=-90
  Saturation1 : Saturate  UpperLimit=30  LowerLimit=-30
  Sum : Sum  Inputs=|+-
  delta_e : Outport
  wires:
  Saturation/1 -> Integrator/1
  Sum/1 -> Gain/1
  Integrator/1 -> Saturation1/1, Sum/2
  delta_e_d/1 -> Sum/1
  Gain/1 -> Saturation/1
  Saturation1/1 -> delta_e/1

== system Ctrl_For_HRV_20260625/Vehicle_2/actuator2_v2 ==
  delta_r_d : Inport
  Gain : Gain  Gain=50
  Integrator : Integrator
  Saturation : Saturate  UpperLimit=90  LowerLimit=-90
  Saturation1 : Saturate  UpperLimit=30  LowerLimit=-30
  Sum : Sum  Inputs=|+-
  delta_r : Outport
  wires:
  Saturation1/1 -> delta_r/1
  Gain/1 -> Saturation/1
  delta_r_d/1 -> Sum/1
  Integrator/1 -> Sum/2, Saturation1/1
  Sum/1 -> Gain/1
  Saturation/1 -> Integrator/1

== system Ctrl_For_HRV_20260625/Vehicle_2/actuator_v2 ==
  delta_a_d : Inport
  Gain : Gain  Gain=50
  Integrator : Integrator
  Saturation : Saturate  UpperLimit=90  LowerLimit=-90
  Saturation1 : Saturate  UpperLimit=30  LowerLimit=-30
  Sum : Sum  Inputs=|+-
  delta_a : Outport
  wires:
  Saturation1/1 -> delta_a/1
  Gain/1 -> Saturation/1
  delta_a_d/1 -> Sum/1
  Integrator/1 -> Sum/2, Saturation1/1
  Sum/1 -> Gain/1
  Saturation/1 -> Integrator/1

== system Ctrl_For_HRV_20260625/Vehicle_3/AngleRate_Controller_v3 ==
  p_d : Inport
  q_d : Inport  Port=2
  r_d : Inport  Port=3
  Demux : Demux  Outputs=9
  Interpreted MATLAB Function : MATLABFcn  MATLABFcn=CCI_DUI_AngleRate_Controller(u(1),u(2),u(3),u(4),u(5),u(6),u(7),u(8),u(9),u(10),u(11),u(12),u(13),u(14),u(15),u(16),u(17),u(18),u(19),u(20),u(21),u(22),u(23))  OutputDimensions=9
  Mux : Mux  Inputs=23
  Mux1 : Mux  Inputs=3
  Mux2 : Mux  Inputs=3
  Scope2 : Scope
  Scope_CCI_AngleRate : Scope
  Scope_DUI_AngleRate : Scope
  Scope_p_d : Scope
  Scope_q_d : Scope
  Scope_r_d : Scope
  TD_p : Subsystem
  TD_q : Subsystem
  TD_r : Subsystem
  delta_a_d : Outport
  delta_e_d : Outport  Port=2
  delta_r_d : Outport  Port=3
  tag scope: delta_a_d_v3=global, delta_e_d_v3=global, delta_r_d_v3=global, p_c_v3=global, q_c_v3=global, r_c_v3=global
  wires:
  Mux2/1 -> Scope_DUI_AngleRate/1
  Demux/9 -> Mux2/3
  Demux/8 -> Mux2/2
  Demux/7 -> Mux2/1
  Mux1/1 -> Scope_CCI_AngleRate/1
  Demux/6 -> Mux1/3
  Demux/5 -> Mux1/2
  Demux/4 -> Mux1/1
  [miu_c_v3] -> Mux/23
  [beta_c_v3] -> Mux/22
  [alpha_c_v3] -> Mux/21
  [phi_r_hat_v3] -> Mux/14
  [phi_q_hat_v3] -> Mux/13
  [phi_p_hat_v3] -> Mux/12
  p_d/1 -> TD_p/1(p_d), Scope_p_d/1
  q_d/1 -> TD_q/1(q_d), Scope_q_d/1
  Demux/1 -> delta_a_d/1, [delta_a_d_v3]
  Demux/2 -> delta_e_d/1, [delta_e_d_v3]
  r_d/1 -> TD_r/1(r_d), Scope_r_d/1
  Demux/3 -> [delta_r_d_v3], delta_r_d/1
  TD_p/1(p_c) -> Mux/15, [p_c_v3]
  [delta_e_v3] -> Mux/7
  [delta_r_v3] -> Mux/8
  [delta_a_v3] -> Mux/6
  Interpreted MATLAB Function/1 -> Demux/1
  Mux/1 -> Interpreted MATLAB Function/1
  [alpha_noise_v3] -> Mux/3
  [V_v3] -> Mux/2
  [p_noise_v3] -> Mux/9
  [H_v3] -> Mux/1
  [r_noise_v3] -> Mux/11
  TD_r/2(r_c_dot) -> Mux/20
  TD_q/1(q_c) -> Mux/17, [q_c_v3]
  [q_noise_v3] -> Mux/10
  TD_q/2(q_c_dot) -> Mux/18
  TD_p/2(p_c_dot) -> Mux/16
  TD_r/1(r_c) -> Mux/19, [r_c_v3]
  [beta_noise_v3] -> Mux/4
  [miu_noise_v3] -> Mux/5

== system Ctrl_For_HRV_20260625/Vehicle_3/AngleRate_ESO_v3 ==
  Add{,1..5} (6 alike) : Sum  Inputs=+-
  Demux : Demux  Outputs=6
  Mux{,1..5} (6 alike) : Mux  Inputs=2
  Mux10 : Mux  Inputs=6
  S-Function : S-Function  FunctionName=fastloop_ESO  SFunctionDeploymentMode=off  EnableBusSupport=off
  Scope_p_hat : Scope
  Scope_p_hat_error : Scope
  Scope_phi_p_hat : Scope
  Scope_phi_p_hat_error : Scope
  Scope_phi_q_hat : Scope
  Scope_phi_q_hat_error : Scope
  Scope_phi_r_hat : Scope
  Scope_phi_r_hat_error : Scope
  Scope_q_hat : Scope
  Scope_q_hat_error : Scope
  Scope_r_hat : Scope
  Scope_r_hat_error : Scope
  tag scope: p_hat_v3=global, phi_p_hat_v3=global, phi_q_hat_v3=global, phi_r_hat_v3=global, q_hat_v3=global, r_hat_v3=global
  wires:
  Add5/1 -> Scope_phi_r_hat_error/1
  [phi_r_hat_v3] -> Add5/2
  [phi_r_v3] -> Add5/1
  Add4/1 -> Scope_phi_q_hat_error/1
  [phi_q_hat_v3] -> Add4/2
  [phi_q_v3] -> Add4/1
  Add3/1 -> Scope_phi_p_hat_error/1
  [phi_p_hat_v3] -> Add3/2
  [phi_p_v3] -> Add3/1
  Add2/1 -> Scope_r_hat_error/1
  [r_hat_v3] -> Add2/2
  [r_noise_v3] -> Add2/1
  Add1/1 -> Scope_q_hat_error/1
  [q_hat_v3] -> Add1/2
  [q_noise_v3] -> Add1/1
  Add/1 -> Scope_p_hat_error/1
  [p_hat_v3] -> Add/2
  [p_noise_v3] -> Add/1
  Mux3/1 -> Scope_phi_p_hat/1
  [phi_p_v3] -> Mux3/1
  [phi_p_hat_v3] -> Mux3/2
  [phi_q_v3] -> Mux4/1
  [phi_q_hat_v3] -> Mux4/2
  Mux4/1 -> Scope_phi_q_hat/1
  [phi_r_v3] -> Mux5/1
  [phi_r_hat_v3] -> Mux5/2
  Mux5/1 -> Scope_phi_r_hat/1
  Mux2/1 -> Scope_r_hat/1
  [r_hat_v3] -> Mux2/2
  [r_noise_v3] -> Mux2/1
  Mux1/1 -> Scope_q_hat/1
  [q_hat_v3] -> Mux1/2
  [q_noise_v3] -> Mux1/1
  [p_hat_v3] -> Mux/2
  [p_noise_v3] -> Mux/1
  Mux/1 -> Scope_p_hat/1
  [b_r_v3] -> Mux10/6
  [p_noise_v3] -> Mux10/1
  Demux/6 -> [phi_r_hat_v3]
  Mux10/1 -> S-Function/1
  Demux/4 -> [phi_p_hat_v3]
  Demux/3 -> [r_hat_v3]
  Demux/1 -> [p_hat_v3]
  Demux/5 -> [phi_q_hat_v3]
  S-Function/1 -> Demux/1
  [b_p_v3] -> Mux10/4
  Demux/2 -> [q_hat_v3]
  [q_noise_v3] -> Mux10/2
  [r_noise_v3] -> Mux10/3
  [b_q_v3] -> Mux10/5

== system Ctrl_For_HRV_20260625/Vehicle_3/Error_Model ==
  Delay : Delay  DelayLength=1
  Delay1 : Delay  DelayLength=1
  Delay2 : Delay  DelayLength=1
  Demux : Demux  Outputs=9
  Mux : Mux  Inputs=33
  S-Function : S-Function  FunctionName=Error_Model  SFunctionDeploymentMode=off  EnableBusSupport=off
  TD_alpha1 : Subsystem
  TD_alpha2 : Subsystem
  TD_alpha3 : Subsystem
  tag scope: dot_e_wd_1=global, dot_e_wd_2=global, dot_e_wd_3=global, e_alpha=global, e_beta=global, e_miu=global, e_w_1=global, e_w_2=global, e_w_3=global, e_wd_1=global, e_wd_2=global, e_wd_3=global
  wires:
  [theta] -> Mux/33
  [r] -> Mux/32
  [q] -> Mux/31
  [p] -> Mux/30
  [miu] -> Mux/29
  [beta] -> Mux/28
  [alpha] -> Mux/27
  [delta_r] -> Mux/3
  [delta_e] -> Mux/2
  [delta_a] -> Mux/1
  [dot_e_wd_3] -> Mux/26
  [dot_e_wd_2] -> Mux/25
  [dot_e_wd_1] -> Mux/24
  TD_alpha3/1(dot_e_wd_3) -> [dot_e_wd_3]
  [e_wd_3] -> TD_alpha3/1(e_wd_3)
  [e_wd_2] -> TD_alpha2/1(e_wd_2)
  TD_alpha2/1(dot_e_wd_2) -> [dot_e_wd_2]
  TD_alpha1/1(dot_e_wd_1) -> [dot_e_wd_1]
  [e_wd_1] -> TD_alpha1/1(e_wd_1)
  Delay2/1 -> Mux/23
  [e_wd_3] -> Delay2/1
  [e_wd_2] -> Delay1/1
  Delay1/1 -> Mux/22
  Delay/1 -> Mux/21
  [e_wd_1] -> Delay/1
  Demux/7 -> [e_wd_1]
  Demux/8 -> [e_wd_2]
  Demux/9 -> [e_wd_3]
  Demux/6 -> [e_w_3]
  Demux/5 -> [e_w_2]
  Demux/4 -> [e_w_1]
  Demux/3 -> [e_miu]
  Demux/2 -> [e_beta]
  Demux/1 -> [e_alpha]
  S-Function/1 -> Demux/1
  [ddot_miu_c] -> Mux/20
  [ddot_beta_c] -> Mux/19
  [ddot_alpha_c] -> Mux/18
  [dot_alpha_c] -> Mux/15
  [dot_beta_c] -> Mux/16
  [dot_miu_c] -> Mux/17
  [miu_c] -> Mux/14
  [beta_c] -> Mux/13
  [alpha_c] -> Mux/12
  [V] -> Mux/11
  [H] -> Mux/10
  [C_m_d] -> Mux/8
  [C_n_d] -> Mux/9
  [C_Y_d] -> Mux/6
  [C_L_d] -> Mux/4
  [C_D_d] -> Mux/5
  [C_l_d] -> Mux/7
  Mux/1 -> S-Function/1

== system Ctrl_For_HRV_20260625/Vehicle_3/FlowAngle_Controller_v3 ==
  alpha_d : Inport
  beta_d : Inport  Port=2
  miu_d : Inport  Port=3
  Demux : Demux  Outputs=9
  From12 : From  Commented=on  GotoTag=dot_alpha_c  TagVisibility=global
  From13 : From  Commented=on  GotoTag=dot_beta_c  TagVisibility=global
  From14 : From  Commented=on  GotoTag=dot_miu_c  TagVisibility=global
  Goto6 : Goto  Commented=on  GotoTag=ddot_alpha_c  TagVisibility=global
  Goto7 : Goto  Commented=on  GotoTag=ddot_beta_c  TagVisibility=global
  Goto8 : Goto  Commented=on  GotoTag=ddot_miu_c  TagVisibility=global
  Interpreted MATLAB Function : MATLABFcn  MATLABFcn=CCI_DUI_FlowAngle_Controller(u(1),u(2),u(3),u(4),u(5),u(6),u(7),u(8),u(9),u(10),u(11),u(12),u(13),u(14),u(15),u(16),u(17),u(18))  OutputDimensions=9
  Mux : Mux  Inputs=18
  Mux1 : Mux  Inputs=3
  Mux2 : Mux  Inputs=3
  Scope_CCI_FlowAngle : Scope
  Scope_DUI_FlowAngle : Scope
  Scope_alpha_d : Scope
  Scope_beta_d : Scope
  Scope_miu_d : Scope
  TD_alpha : Subsystem
  TD_alpha2 : Subsystem
  TD_alpha3 : Subsystem  Commented=on
  TD_alpha4 : Subsystem  Commented=on
  TD_beta : Subsystem
  TD_beta1 : Subsystem
  TD_beta2 : Subsystem
  TD_dotalpha1 : Subsystem  Commented=on
  TD_miu : Subsystem
  p_d : Outport
  q_d : Outport  Port=2
  r_d : Outport  Port=3
  tag scope: alpha_c_v3=global, beta_c_v3=global, dot_alpha_c_v3=global, dot_beta_c_v3=global, dot_miu_c_v3=global, miu_c_v3=global
  wires:
  Demux/7 -> Mux2/1
  Demux/9 -> Mux2/3
  Demux/8 -> Mux2/2
  Mux2/1 -> Scope_DUI_FlowAngle/1
  Mux1/1 -> Scope_CCI_FlowAngle/1
  Demux/6 -> Mux1/3
  Demux/5 -> Mux1/2
  Demux/4 -> Mux1/1
  TD_alpha/1(alpha_c) -> Mux/13, [alpha_c_v3]
  TD_alpha4/1(ddot_miu_c) -> Goto8/1
  From14/1 -> TD_alpha4/1(dot_miu_c)
  TD_alpha3/1(ddot_beta_c) -> Goto7/1
  From13/1 -> TD_alpha3/1(dot_beta_c)
  TD_dotalpha1/1(ddot_alpha_c) -> Goto6/1
  From12/1 -> TD_dotalpha1/1(dot_alpha_c)
  [phi_miu_hat_v3] -> Mux/12
  [phi_beta_hat_v3] -> Mux/11
  [phi_alpha_hat_v3] -> Mux/10
  TD_miu/2(miu_c_dot) -> Mux/18, [dot_miu_c_v3]
  TD_miu/1(miu_c) -> Mux/17, [miu_c_v3]
  miu_d/1 -> TD_miu/1(miu_d), Scope_miu_d/1
  TD_beta/2(beta_c_dot) -> Mux/16, [dot_beta_c_v3]
  TD_beta/1(beta_c) -> Mux/15, [beta_c_v3]
  beta_d/1 -> TD_beta/1(beta_d), Scope_beta_d/1
  TD_alpha/2(alpha_c_dot) -> [dot_alpha_c_v3], Mux/14
  alpha_d/1 -> TD_alpha/1(alpha_d), Scope_alpha_d/1
  Demux/3 -> r_d/1
  Demux/2 -> q_d/1
  Demux/1 -> p_d/1
  Interpreted MATLAB Function/1 -> Demux/1
  Mux/1 -> Interpreted MATLAB Function/1
  [theta_v3] -> Mux/9
  [delta_a_v3] -> Mux/6
  [delta_e_v3] -> Mux/7
  [delta_r_v3] -> Mux/8
  [miu_noise_v3] -> Mux/5
  [beta_noise_v3] -> Mux/4
  [alpha_noise_v3] -> Mux/3
  [V_v3] -> Mux/2
  [H_v3] -> Mux/1

== system Ctrl_For_HRV_20260625/Vehicle_3/FlowAngle_ESO_v3 ==
  Add{,1..5} (6 alike) : Sum  Inputs=+-
  Demux : Demux  Outputs=6
  Mux{,1..5} (6 alike) : Mux  Inputs=2
  Mux10 : Mux  Inputs=6
  S-Function : S-Function  FunctionName=slowloop_ESO  SFunctionDeploymentMode=off  EnableBusSupport=off
  Scope_alpha_hat : Scope
  Scope_alpha_hat_error : Scope
  Scope_beta_hat : Scope
  Scope_beta_hat_error : Scope
  Scope_miu_hat : Scope
  Scope_miu_hat_error : Scope
  Scope_phi_alpha_hat : Scope
  Scope_phi_alpha_hat_error : Scope
  Scope_phi_beta_hat : Scope
  Scope_phi_beta_hat_error : Scope
  Scope_phi_miu_hat : Scope
  Scope_phi_miu_hat_error : Scope
  tag scope: alpha_hat_v3=global, beta_hat_v3=global, miu_hat_v3=global, phi_alpha_hat_v3=global, phi_beta_hat_v3=global, phi_miu_hat_v3=global
  wires:
  [phi_miu_hat_v3] -> Add5/2
  [phi_miu_v3] -> Add5/1
  Add5/1 -> Scope_phi_miu_hat_error/1
  Add4/1 -> Scope_phi_beta_hat_error/1
  [phi_beta_hat_v3] -> Add4/2
  [phi_beta_v3] -> Add4/1
  Add3/1 -> Scope_phi_alpha_hat_error/1
  [phi_alpha_hat_v3] -> Add3/2
  [phi_alpha_v3] -> Add3/1
  Add2/1 -> Scope_miu_hat_error/1
  [miu_hat_v3] -> Add2/2
  [miu_noise_v3] -> Add2/1
  Add1/1 -> Scope_beta_hat_error/1
  [beta_hat_v3] -> Add1/2
  [beta_noise_v3] -> Add1/1
  Add/1 -> Scope_alpha_hat_error/1
  [alpha_hat_v3] -> Add/2
  [alpha_noise_v3] -> Add/1
  Mux3/1 -> Scope_phi_alpha_hat/1
  [phi_alpha_v3] -> Mux3/1
  [phi_alpha_hat_v3] -> Mux3/2
  [phi_beta_v3] -> Mux4/1
  [phi_beta_hat_v3] -> Mux4/2
  Mux4/1 -> Scope_phi_beta_hat/1
  [phi_miu_v3] -> Mux5/1
  [phi_miu_hat_v3] -> Mux5/2
  Mux5/1 -> Scope_phi_miu_hat/1
  Mux2/1 -> Scope_miu_hat/1
  [miu_hat_v3] -> Mux2/2
  [miu_noise_v3] -> Mux2/1
  Mux1/1 -> Scope_beta_hat/1
  [beta_hat_v3] -> Mux1/2
  [beta_noise_v3] -> Mux1/1
  [alpha_hat_v3] -> Mux/2
  [alpha_noise_v3] -> Mux/1
  Mux/1 -> Scope_alpha_hat/1
  [b_miu_v3] -> Mux10/6
  [alpha_noise_v3] -> Mux10/1
  Demux/6 -> [phi_miu_hat_v3]
  Mux10/1 -> S-Function/1
  Demux/4 -> [phi_alpha_hat_v3]
  Demux/3 -> [miu_hat_v3]
  Demux/1 -> [alpha_hat_v3]
  Demux/5 -> [phi_beta_hat_v3]
  S-Function/1 -> Demux/1
  [b_alpha_v3] -> Mux10/4
  Demux/2 -> [beta_hat_v3]
  [beta_noise_v3] -> Mux10/2
  [miu_noise_v3] -> Mux10/3
  [b_beta_v3] -> Mux10/5

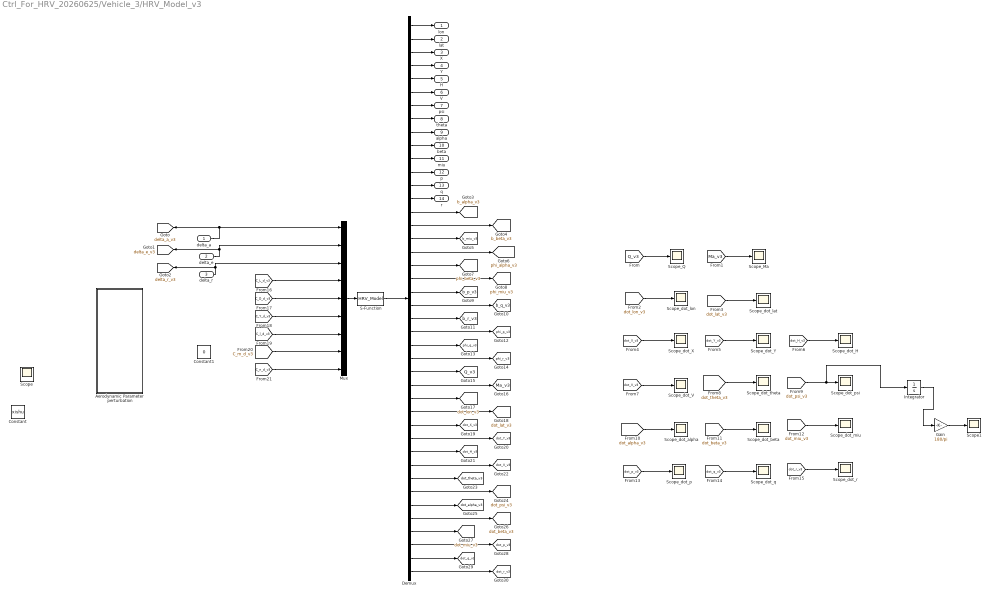
== system Ctrl_For_HRV_20260625/Vehicle_3/HRV_Model_v3 ==
  delta_a : Inport
  delta_e : Inport  Port=2
  delta_r : Inport  Port=3
  Aerodynamic Parameter perturbation : Subsystem
  Constant : Constant  Value=xishu  SampleTime=-1
  Constant1 : Constant  Value=0
  Demux : Demux  Outputs=14 + 12 + 2 + 14
  Gain : Gain  Gain=180/pi
  Integrator : Integrator  InitialCondition=[0 0 0 0 0 0 0 0 0 0 0 0 0 0 0 0 0 0 0 0 0 0 0 0 0 0 0 0 0 0 0 0 0 0 0 0 0 0 0 0 0 0]
  Mux : Mux  Inputs=9
  S-Function : S-Function  FunctionName=HRV_Model  SFunctionDeploymentMode=off  EnableBusSupport=off
  Scope : Scope
  Scope1 : Scope
  Scope_Ma : Scope
  Scope_Q : Scope
  Scope_dot_H : Scope
  Scope_dot_V : Scope
  Scope_dot_X : Scope
  Scope_dot_Y : Scope
  Scope_dot_alpha : Scope
  Scope_dot_beta : Scope
  Scope_dot_lat : Scope
  Scope_dot_lon : Scope
  Scope_dot_miu : Scope
  Scope_dot_p : Scope
  Scope_dot_psi : Scope
  Scope_dot_q : Scope
  Scope_dot_r : Scope
  Scope_dot_theta : Scope
  lon : Outport
  lat : Outport  Port=2
  X : Outport  Port=3
  Y : Outport  Port=4
  H : Outport  Port=5
  V : Outport  Port=6
  psi : Outport  Port=7
  theta : Outport  Port=8
  alpha : Outport  Port=9
  beta : Outport  Port=10
  miu : Outport  Port=11
  p : Outport  Port=12
  q : Outport  Port=13
  r : Outport  Port=14
  tag scope: Ma_v3=global, Q_v3=global, b_alpha_v3=global, b_beta_v3=global, b_miu_v3=global, b_p_v3=global, b_q_v3=global, b_r_v3=global, delta_a_v3=global, delta_e_v3=global, delta_r_v3=global, dot_H_v3=global, dot_V_v3=global, dot_X_v3=global, dot_Y_v3=global, dot_alpha_v3=global, dot_beta_v3=global, dot_lat_v3=global, dot_lon_v3=global, dot_miu_v3=global, dot_p_v3=global, dot_psi_v3=global, dot_q_v3=global, dot_r_v3=global, dot_theta_v3=global, phi_alpha_v3=global, phi_beta_v3=global, phi_miu_v3=global, phi_p_v3=global, phi_q_v3=global, phi_r_v3=global
  wires:
  Gain/1 -> Scope1/1
  Integrator/1 -> Gain/1
  [C_n_d_v3] -> Mux/9
  [C_m_d_v3] -> Mux/8
  [C_l_d_v3] -> Mux/7
  [C_Y_d_v3] -> Mux/6
  [C_D_d_v3] -> Mux/5
  [C_L_d_v3] -> Mux/4
  [dot_p_v3] -> Scope_dot_p/1
  [dot_q_v3] -> Scope_dot_q/1
  [dot_r_v3] -> Scope_dot_r/1
  [dot_miu_v3] -> Scope_dot_miu/1
  [dot_beta_v3] -> Scope_dot_beta/1
  [dot_alpha_v3] -> Scope_dot_alpha/1
  [dot_psi_v3] -> Scope_dot_psi/1, Integrator/1
  [dot_theta_v3] -> Scope_dot_theta/1
  [dot_V_v3] -> Scope_dot_V/1
  [dot_H_v3] -> Scope_dot_H/1
  [dot_Y_v3] -> Scope_dot_Y/1
  [dot_X_v3] -> Scope_dot_X/1
  [dot_lat_v3] -> Scope_dot_lat/1
  [dot_lon_v3] -> Scope_dot_lon/1
  [Ma_v3] -> Scope_Ma/1
  [Q_v3] -> Scope_Q/1
  Demux/42 -> [dot_r_v3]
  Demux/41 -> [dot_q_v3]
  Demux/40 -> [dot_p_v3]
  Demux/38 -> [dot_beta_v3]
  Demux/39 -> [dot_miu_v3]
  Demux/33 -> [dot_H_v3]
  Demux/35 -> [dot_theta_v3]
  Demux/34 -> [dot_V_v3]
  Demux/36 -> [dot_psi_v3]
  Demux/37 -> [dot_alpha_v3]
  Demux/32 -> [dot_Y_v3]
  Demux/31 -> [dot_X_v3]
  Demux/29 -> [dot_lon_v3]
  Demux/30 -> [dot_lat_v3]
  Demux/28 -> [Ma_v3]
  Demux/27 -> [Q_v3]
  Demux/26 -> [phi_r_v3]
  Demux/25 -> [phi_q_v3]
  Demux/24 -> [phi_p_v3]
  Demux/23 -> [b_r_v3]
  Demux/19 -> [phi_beta_v3]
  Demux/20 -> [phi_miu_v3]
  Demux/22 -> [b_q_v3]
  Demux/21 -> [b_p_v3]
  Demux/17 -> [b_miu_v3]
  Demux/18 -> [phi_alpha_v3]
  Demux/16 -> [b_beta_v3]
  Demux/15 -> [b_alpha_v3]
  Demux/4 -> Y/1
  delta_a/1 -> Mux/1, [delta_a_v3]
  Demux/13 -> q/1
  delta_r/1 -> Mux/3, [delta_r_v3]
  Demux/14 -> r/1
  Demux/6 -> V/1
  delta_e/1 -> Mux/2, [delta_e_v3]
  Demux/5 -> H/1
  Demux/12 -> p/1
  Demux/9 -> alpha/1
  Demux/10 -> beta/1
  Demux/11 -> miu/1
  Demux/7 -> psi/1
  Demux/3 -> X/1
  Demux/2 -> lat/1
  Demux/1 -> lon/1
  S-Function/1 -> Demux/1
  Mux/1 -> S-Function/1
  Demux/8 -> theta/1

== system Ctrl_For_HRV_20260625/Vehicle_3/PNG ==
  Delay : Delay  DelayLength=1
  Demux : Demux  Outputs=3
  MATLAB Function : MATLAB Function  TreatAsAtomicUnit=on
  MATLAB Function1 : MATLAB Function  TreatAsAtomicUnit=on  SystemSampleTime=0.02
  MATLAB Function2 : MATLAB Function  TreatAsAtomicUnit=on
  Mux : Mux  Inputs=7+2
  PNG : MATLABFcn  MATLABFcn=PNG_2026_6_23(u)  OutputDimensions=3
  Scope{,1..4} (5 alike) : Scope
  Scope5 : Scope  NumInputPorts=2
  tag scope: alpha_cmd=global, f_psi=global, miu_cmd=global
  wires:
  Delay/1 -> MATLAB Function1/6(miu_last)
  [theta] -> Mux/9
  [f_psi] -> Mux/8
  MATLAB Function2/1(f_psi) -> [f_psi]
  [H] -> MATLAB Function2/5(H)
  [lat] -> MATLAB Function2/4(lat)
  [psi] -> MATLAB Function2/3(psi)
  [theta] -> MATLAB Function2/2(theta)
  [V] -> MATLAB Function2/1(V)
  Demux/3 -> Scope5/1
  [Q] -> Mux/7
  MATLAB Function1/2(miu_cmd) -> [miu_cmd], Scope3/1, Delay/1
  MATLAB Function1/1(alpha_cmd) -> [alpha_cmd], Scope2/1
  [Ma] -> MATLAB Function1/5(Ma)
  [H] -> MATLAB Function1/4(H)
  [Q] -> MATLAB Function1/3(Q)
  [nz_cmd] -> MATLAB Function1/2(nz_cmd)
  [ny_cmd] -> MATLAB Function1/1(ny_cmd)
  [nz_cmd] -> Scope1/1
  [ny_cmd] -> Scope/1
  Demux/2 -> [nz_cmd], Scope5/2
  Demux/1 -> [ny_cmd]
  PNG/1 -> Demux/1
  [V_target] -> Mux/6
  [Position_target] -> Mux/5
  MATLAB Function/1(v) -> Mux/4, Scope4/1
  [psi] -> MATLAB Function/3(psi)
  [theta] -> MATLAB Function/2(theta)
  [V] -> MATLAB Function/1(V)
  [H] -> Mux/3
  [Y] -> Mux/2
  [X] -> Mux/1
  Mux/1 -> PNG/1

== system Ctrl_For_HRV_20260625/Vehicle_3/actuator1_v3 ==
  delta_e_d : Inport
  Gain : Gain  Gain=50
  Integrator : Integrator
  Saturation : Saturate  UpperLimit=90  LowerLimit=-90
  Saturation1 : Saturate  UpperLimit=30  LowerLimit=-30
  Sum : Sum  Inputs=|+-
  delta_e : Outport
  wires:
  Saturation/1 -> Integrator/1
  Sum/1 -> Gain/1
  Integrator/1 -> Saturation1/1, Sum/2
  delta_e_d/1 -> Sum/1
  Gain/1 -> Saturation/1
  Saturation1/1 -> delta_e/1

== system Ctrl_For_HRV_20260625/Vehicle_3/actuator2_v3 ==
  delta_r_d : Inport
  Gain : Gain  Gain=50
  Integrator : Integrator
  Saturation : Saturate  UpperLimit=90  LowerLimit=-90
  Saturation1 : Saturate  UpperLimit=30  LowerLimit=-30
  Sum : Sum  Inputs=|+-
  delta_r : Outport
  wires:
  Saturation1/1 -> delta_r/1
  Gain/1 -> Saturation/1
  delta_r_d/1 -> Sum/1
  Integrator/1 -> Sum/2, Saturation1/1
  Sum/1 -> Gain/1
  Saturation/1 -> Integrator/1

== system Ctrl_For_HRV_20260625/Vehicle_3/actuator_v3 ==
  delta_a_d : Inport
  Gain : Gain  Gain=50
  Integrator : Integrator
  Saturation : Saturate  UpperLimit=90  LowerLimit=-90
  Saturation1 : Saturate  UpperLimit=30  LowerLimit=-30
  Sum : Sum  Inputs=|+-
  delta_a : Outport
  wires:
  Saturation1/1 -> delta_a/1
  Gain/1 -> Saturation/1
  delta_a_d/1 -> Sum/1
  Integrator/1 -> Sum/2, Saturation1/1
  Sum/1 -> Gain/1
  Saturation/1 -> Integrator/1

== system Ctrl_For_HRV_20260625/Vehicle_4/AngleRate_Controller_v4 ==
  p_d : Inport
  q_d : Inport  Port=2
  r_d : Inport  Port=3
  Demux : Demux  Outputs=9
  Interpreted MATLAB Function : MATLABFcn  MATLABFcn=CCI_DUI_AngleRate_Controller(u(1),u(2),u(3),u(4),u(5),u(6),u(7),u(8),u(9),u(10),u(11),u(12),u(13),u(14),u(15),u(16),u(17),u(18),u(19),u(20),u(21),u(22),u(23))  OutputDimensions=9
  Mux : Mux  Inputs=23
  Mux1 : Mux  Inputs=3
  Mux2 : Mux  Inputs=3
  Scope2 : Scope
  Scope_CCI_AngleRate : Scope
  Scope_DUI_AngleRate : Scope
  Scope_p_d : Scope
  Scope_q_d : Scope
  Scope_r_d : Scope
  TD_p : Subsystem
  TD_q : Subsystem
  TD_r : Subsystem
  delta_a_d : Outport
  delta_e_d : Outport  Port=2
  delta_r_d : Outport  Port=3
  tag scope: delta_a_d_v4=global, delta_e_d_v4=global, delta_r_d_v4=global, p_c_v4=global, q_c_v4=global, r_c_v4=global
  wires:
  Mux2/1 -> Scope_DUI_AngleRate/1
  Demux/9 -> Mux2/3
  Demux/8 -> Mux2/2
  Demux/7 -> Mux2/1
  Mux1/1 -> Scope_CCI_AngleRate/1
  Demux/6 -> Mux1/3
  Demux/5 -> Mux1/2
  Demux/4 -> Mux1/1
  [miu_c_v4] -> Mux/23
  [beta_c_v4] -> Mux/22
  [alpha_c_v4] -> Mux/21
  [phi_r_hat_v4] -> Mux/14
  [phi_q_hat_v4] -> Mux/13
  [phi_p_hat_v4] -> Mux/12
  p_d/1 -> TD_p/1(p_d), Scope_p_d/1
  q_d/1 -> TD_q/1(q_d), Scope_q_d/1
  Demux/1 -> delta_a_d/1, [delta_a_d_v4]
  Demux/2 -> delta_e_d/1, [delta_e_d_v4]
  r_d/1 -> TD_r/1(r_d), Scope_r_d/1
  Demux/3 -> [delta_r_d_v4], delta_r_d/1
  TD_p/1(p_c) -> Mux/15, [p_c_v4]
  [delta_e_v4] -> Mux/7
  [delta_r_v4] -> Mux/8
  [delta_a_v4] -> Mux/6
  Interpreted MATLAB Function/1 -> Demux/1
  Mux/1 -> Interpreted MATLAB Function/1
  [alpha_noise_v4] -> Mux/3
  [V_v4] -> Mux/2
  [p_noise_v4] -> Mux/9
  [H_v4] -> Mux/1
  [r_noise_v4] -> Mux/11
  TD_r/2(r_c_dot) -> Mux/20
  TD_q/1(q_c) -> Mux/17, [q_c_v4]
  [q_noise_v4] -> Mux/10
  TD_q/2(q_c_dot) -> Mux/18
  TD_p/2(p_c_dot) -> Mux/16
  TD_r/1(r_c) -> Mux/19, [r_c_v4]
  [beta_noise_v4] -> Mux/4
  [miu_noise_v4] -> Mux/5
